simulink model "FlowChart_PedalPositionSensor"  (R2024a)
settings: Solver=VariableStepAuto  StartTime=0.0  StopTime=10.0  RelTol=1e-3
settings Model: Creator=VICTUS  LastModifiedBy=VICTUS

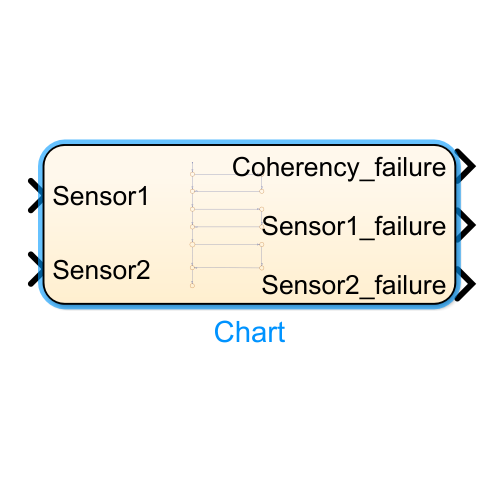
[thumbnail: Simulink's stored preview of the top-level diagram]
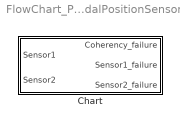
== system FlowChart_PedalPositionSensor ==
  Chart : Stateflow chart  TreatAsAtomicUnit=on

== stateflow chart FlowChart_PedalPositionSensor/Chart ==
  (default) -> (junction 1)
  (junction 1) -> (junction 3) [order 1] : [Sensor1 >4.5 || Sensor1 < 0.5]
  (junction 1) -> (junction 7) [order 2]
  (junction 3) -> (junction 5) : {Sensor1_failure = 1;}
  (junction 5) -> (junction 7)
  (junction 7) -> (junction 20)
  (junction 20) -> (junction 16) [order 1] : [Sensor2 >4.5 || Sensor2 <0.5]
  (junction 20) -> (junction 25) [order 2]
  (junction 16) -> (junction 23) : {Sensor2_failure = 1;}
  (junction 23) -> (junction 25)
  (junction 25) -> (junction 38)
  (junction 38) -> (junction 35) [order 1] : [Sensor1+Sensor2 ~= 5]
  (junction 35) -> (junction 40) : {Coherency_failure = 1;}
  (junction 38) -> (junction 43) [order 2]
  (junction 40) -> (junction 43)
  (junction 43) -> (junction 59)
  data: Sensor1 input double; Sensor2 input double; Coherency_failure output boolean; Sensor1_failure output boolean; Sensor2_failure output boolean
